simulink model "Miss_Sim_MatrixPilot"  (Simulink 7.0)
settings: Solver=ode1  SolverMode=SingleTasking  StartTime=0.0  StopTime=120  FixedStep=0.00025  MaxStep=0.01  MinStep=0.000001  RelTol=1e-12  AbsTol=1e-12
values from neighbouring files (symbols this model uses):
  alpha = [-180.     -90.        -5.         0.         5.        10.        15.        90.       180.       ]    [Miss_Data.m]
  Bref = 1.4    [Miss_Data.m]
  Clail = [ 0.         0.         0.         0.         0.         0.         0.         0.         0.       ]    [Miss_Data.m]
  Clp = [-0.5000    -0.5000    -0.496303  -0.494610  -0.492441  -0.492625  -0.522141  -0.5000    -0.5000   ]    [Miss_Data.m]
  Clr = [ 0.         0.         0.064175   0.123689   0.182593   0.241565   0.304725   0.         0.       ]    [Miss_Data.m]
  Clrud = [-0.000045  -0.000045  -0.000051  -0.000049  -0.000047  -0.000043  -0.000039  -0.000045  -0.000045 ]    [Miss_Data.m]
  Clv = [ 0.         0.        -0.098934  -0.137639  -0.176627  -0.217863  -0.281334   0.         0.       ]    [Miss_Data.m]
  Cmele = [-0.0180    -0.0180    -0.019125  -0.019236  -0.019052  -0.018576  -0.017796  -0.0180    -0.0180   ]    [Miss_Data.m]
  Cmq = [-12.3     -12.3      -12.288971 -12.358734 -12.331396 -12.223111 -12.072741 -12.3      -12.3      ]    [Miss_Data.m]
  Cmtot = [ 0.         2.         0.097340   0.036740  -0.047230  -0.137480  -0.110880  -2.         0.       ]    [Miss_Data.m]
  Cnail = [ 0.         0.         0.         0.         0.         0.         0.         0.         0.       ]    [Miss_Data.m]
  Cnp = [ 0.         0.         0.027830  -0.031473  -0.087981  -0.137950  -0.158851   0.         0.       ]    [Miss_Data.m]
  Cnr = [ 0.         0.        -0.041684  -0.040009  -0.043373  -0.056062  -0.120565   0.         0.       ]    [Miss_Data.m]
  Cnrud = [ 0.         0.         0.000628   0.000668   0.000698   0.000717   0.000725   0.         0.       ]    [Miss_Data.m]
  Cnv = [ 0.         0.         0.011072   0.000612  -0.009401  -0.018785  -0.019172   0.         0.       ]    [Miss_Data.m]
  Cref = 0.20    (= 0.2)    [Miss_Data.m]
  CROSS_TRACK = 1    [MatrixPilot_Parameters.m]
  CXq = [ 0.         0.        -0.507981  -0.147630   0.201483   0.570203   1.026474   0.         0.       ]    [Miss_Data.m]
  CXtot = [ 0.03       0.        -0.060470  -0.054540   0.003010   0.075240  -0.109550   0.         0.03     ]    [Miss_Data.m]
  CYp = [ 0.         0.        -0.217329  -0.145848  -0.074905  -0.009210   0.015572   0.         0.       ]    [Miss_Data.m]
  CYr = [ 0.         0.         0.049134   0.076782   0.103755   0.129584   0.152004   0.         0.       ]    [Miss_Data.m]
  CYrud = [-0.0016    -0.0016    -0.001484  -0.001575  -0.001641  -0.001681  -0.001693  -0.0016    -0.0016   ]    [Miss_Data.m]
  CYv = [ 0.         0.        -0.204296  -0.201289  -0.208918  -0.263073  -0.644029   0.         0.       ]    [Miss_Data.m]
  CZele = [-0.0067    -0.0067    -0.006924  -0.006962  -0.006897  -0.006734  -0.006498  -0.0067    -0.0067   ]    [Miss_Data.m]
  CZq = [ 0.         0.        -9.116849  -8.745556  -8.332987  -7.894125  -7.541102   0.         0.       ]    [Miss_Data.m]
  CZtot = [ 0.        10.         0.102580  -0.382550  -0.864940  -1.339340  -1.876430 -10.         0.       ]    [Miss_Data.m]
  DH = 10.    (= 10)    [MatrixPilot_Parameters.m]
  ele_damping = 0.7    [Miss_Data.m]
  ele_def_max = 30.    (= 30)    [Miss_Data.m]
  ele_frequency = 150.    (= 150)    [Miss_Data.m]
  ele_rate_limit = 285.    (= 285)    [Miss_Data.m]
  Ixx = 0.03004    [Miss_Data.m]
  Ixy = 0.    (= 0)    [Miss_Data.m]
  Ixz = 0.00137    [Miss_Data.m]
  Iyx = Ixy    (= 0)    [Miss_Data.m]
  Iyy = 0.01916    [Miss_Data.m]
  Iyz = 0.    (= 0)    [Miss_Data.m]
  Izx = Ixz    (= 0.00137)    [Miss_Data.m]
  Izy = Iyz    (= 0)    [Miss_Data.m]
  Izz = 0.04573    [Miss_Data.m]
  Mass = 0.950    (= 0.95)    [Miss_Data.m]
  rud_damping = 0.7    [Miss_Data.m]
  rud_def_max = 30.    (= 30)    [Miss_Data.m]
  rud_frequency = 150.    (= 150)    [Miss_Data.m]
  rud_rate_limit = 285.    (= 285)    [Miss_Data.m]
  SPEED_CONTROL = 1    [MatrixPilot_Parameters.m]
  Sref = 0.28    [Miss_Data.m]
  T_max = 1.    (= 1)    [MatrixPilot_Parameters.m]
  T_min = 0.35    [MatrixPilot_Parameters.m]
  Tdgps = 1.    (= 1)    [Miss_Data.m]
  theta_0 = -15.    (= -15)    [MatrixPilot_Parameters.m]
  theta_max = 15.    (= 15)    [MatrixPilot_Parameters.m]
  theta_min = -15.    (= -15)    [MatrixPilot_Parameters.m]
  Tmax = 10.    (= 10)    [Miss_Data.m]
  Vsp = 10.    (= 10)    [MatrixPilot_Parameters.m]
  WAYPOINT_RADIUS = 30.    (= 30)    [MatrixPilot_Parameters.m]
undefined symbols (not defined in the file or in its folder): F, MIL, Moderate
libraries: simulink x41, simulink_extras x26, dspstat3 x2, aerospace x1, aerolibanim x1, aerolibwind2 x1
(part 2 of 2)

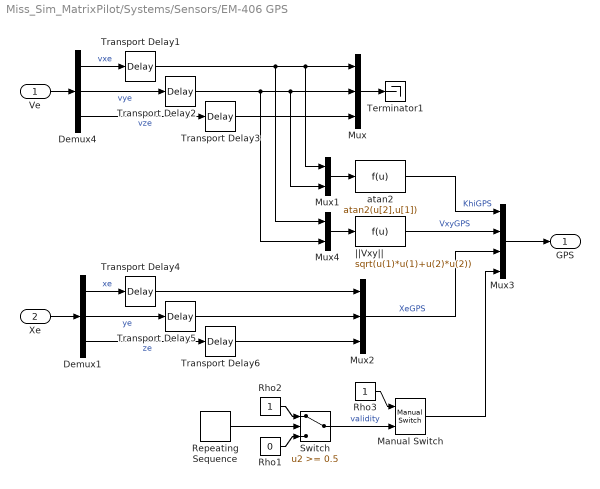
== system Miss_Sim_MatrixPilot/Systems/Sensors/EM-406 GPS ==
  Ve : Inport
  Xe : Inport  Port=2
  Demux1 : Demux  Outputs=3
  Demux4 : Demux  Outputs=3
  Manual Switch : simulink/Signal Routing/Manual Switch  SystemSampleTime=-1  sw=1  action=0  varsize=off
  Mux : Mux  Inputs=3
  Mux1 : Mux  Inputs=2
  Mux2 : Mux  Inputs=3
  Mux3 : Mux
  Mux4 : Mux  Inputs=2
  Repeating Sequence : simulink/Sources/Repeating Sequence  SystemSampleTime=-1  rep_seq_t="[0   120   120.001    140.  140.001  5000]"  rep_seq_y="[1    1       0           0        1          1]"
  Rho1 : Constant  Value=0
  Rho2 : Constant
  Rho3 : Constant
  Switch : Switch  Threshold=0.5  OutDataType=sfix(16)  OutScaling=2^0
  Terminator1 : Terminator
  Transport Delay1 : TransportDelay  DelayTime=Tdgps  InitialOutput=8.  BufferSize=4096
  Transport Delay{2..5} (4 alike) : TransportDelay  DelayTime=Tdgps  BufferSize=4096
  Transport Delay6 : TransportDelay  DelayTime=Tdgps  InitialOutput=-75  BufferSize=4096
  atan2 : Fcn  Expr=atan2(u[2],u[1])
  ||Vxy|| : Fcn  Expr=sqrt(u(1)*u(1)+u(2)*u(2))
  GPS : Outport
  wires:
  Transport Delay6/1 -> Mux2/3
  Transport Delay5/1 -> Mux2/2
  Transport Delay4/1 -> Mux2/1
  Transport Delay3/1 -> Mux/3
  Transport Delay2/1 -> Mux1/2, Mux/2, Mux4/2
  Transport Delay1/1 -> Mux1/1, Mux/1, Mux4/1
  Rho3/1 -> Manual Switch/1
  Manual Switch/1 -> Mux3/4
  Switch/1 -> Manual Switch/2  "validity"
  Repeating Sequence/1 -> Switch/2
  Rho2/1 -> Switch/1
  Rho1/1 -> Switch/3
  Mux3/1 -> GPS/1
  ||Vxy||/1 -> Mux3/2  "VxyGPS"
  Mux4/1 -> ||Vxy||/1
  Demux1/3 -> Transport Delay6/1  "ze"
  Xe/1 -> Demux1/1
  Mux2/1 -> Mux3/3  "XeGPS"
  Demux1/2 -> Transport Delay5/1  "ye"
  Demux1/1 -> Transport Delay4/1  "xe"
  Demux4/3 -> Transport Delay3/1  "vze"
  atan2/1 -> Mux3/1  "KhiGPS"
  Mux1/1 -> atan2/1
  Ve/1 -> Demux4/1
  Mux/1 -> Terminator1/1
  Demux4/2 -> Transport Delay2/1  "vye"
  Demux4/1 -> Transport Delay1/1  "vxe"

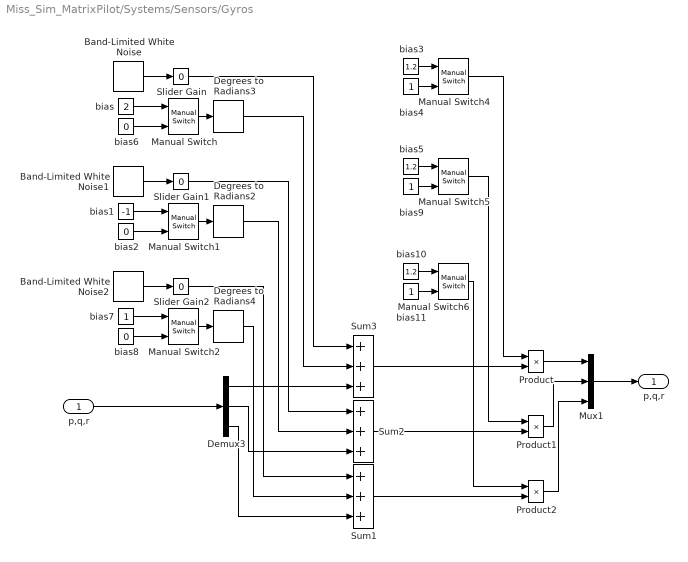
== system Miss_Sim_MatrixPilot/Systems/Sensors/Gyros ==
  p,q,r : Inport
  Band-Limited White Noise : simulink/Sources/Band-Limited White Noise  SystemSampleTime=-1  Cov=[0.000001]  Ts=0.01  seed=[23341]
  Band-Limited White Noise1 : simulink/Sources/Band-Limited White Noise  SystemSampleTime=-1  Cov=[0.000001]  Ts=0.01  seed=[23341]
  Band-Limited White Noise2 : simulink/Sources/Band-Limited White Noise  SystemSampleTime=-1  Cov=[0.000001]  Ts=0.01  seed=[23341]
  Degrees to Radians2 : simulink_extras/Transformations/Degrees to Radians  SystemSampleTime=-1
  Degrees to Radians3 : simulink_extras/Transformations/Degrees to Radians  SystemSampleTime=-1
  Degrees to Radians4 : simulink_extras/Transformations/Degrees to Radians  SystemSampleTime=-1
  Demux3 : Demux  Outputs=3
  Manual Switch{,1..2,4..6} (6 alike) : simulink/Signal Routing/Manual Switch  SystemSampleTime=-1  sw=0  action=0  varsize=off
  Mux1 : Mux  Inputs=3
  Product : Product  SaturateOnIntegerOverflow=on  RndMeth=Zero  InputSameDT=on
  Product1 : Product  SaturateOnIntegerOverflow=on  RndMeth=Zero  InputSameDT=on
  Product2 : Product  SaturateOnIntegerOverflow=on  RndMeth=Zero  InputSameDT=on
  Slider Gain : simulink/Math Operations/Slider Gain  SystemSampleTime=-1  low=0  gain=0  high=2
  Slider Gain1 : simulink/Math Operations/Slider Gain  SystemSampleTime=-1  low=0  gain=0  high=2
  Slider Gain2 : simulink/Math Operations/Slider Gain  SystemSampleTime=-1  low=0  gain=0  high=2
  Sum1 : Sum  Inputs=+++  SaturateOnIntegerOverflow=on  InputSameDT=on
  Sum2 : Sum  Inputs=+++  SaturateOnIntegerOverflow=on  InputSameDT=on
  Sum3 : Sum  Inputs=+++  SaturateOnIntegerOverflow=on  InputSameDT=on
  bias : Constant  Value=2  VectorParams1D=off
  bias1 : Constant  Value=-1  VectorParams1D=off
  bias10 : Constant  Value=1.2  VectorParams1D=off
  bias{4,7,9,11} (4 alike) : Constant  VectorParams1D=off
  bias2 : Constant  Value=0  VectorParams1D=off
  bias3 : Constant  Value=1.2  VectorParams1D=off
  bias5 : Constant  Value=1.2  VectorParams1D=off
  bias6 : Constant  Value=0  VectorParams1D=off
  bias8 : Constant  Value=0  VectorParams1D=off
  "p,q,r " : Outport
  wires:
  Mux1/1 -> "p,q,r "/1
  p,q,r/1 -> Demux3/1
  Band-Limited White Noise/1 -> Slider Gain/1
  Demux3/3 -> Sum1/3
  Demux3/2 -> Sum2/3
  Demux3/1 -> Sum3/3
  Band-Limited White Noise1/1 -> Slider Gain1/1
  Band-Limited White Noise2/1 -> Slider Gain2/1
  Slider Gain2/1 -> Sum1/1
  Slider Gain1/1 -> Sum2/1
  Slider Gain/1 -> Sum3/1
  Sum3/1 -> Product/2
  Product/1 -> Mux1/1
  Sum2/1 -> Product1/2
  Product1/1 -> Mux1/2
  Sum1/1 -> Product2/2
  Product2/1 -> Mux1/3
  Manual Switch4/1 -> Product/1
  Manual Switch6/1 -> Product2/1
  Manual Switch5/1 -> Product1/1
  Degrees to Radians3/1 -> Sum3/2
  Degrees to Radians2/1 -> Sum2/2
  Degrees to Radians4/1 -> Sum1/2
  Manual Switch/1 -> Degrees to Radians3/1
  bias/1 -> Manual Switch/1
  bias6/1 -> Manual Switch/2
  bias1/1 -> Manual Switch1/1
  bias2/1 -> Manual Switch1/2
  bias7/1 -> Manual Switch2/1
  bias8/1 -> Manual Switch2/2
  Manual Switch2/1 -> Degrees to Radians4/1
  Manual Switch1/1 -> Degrees to Radians2/1
  bias3/1 -> Manual Switch4/1
  bias4/1 -> Manual Switch4/2
  bias5/1 -> Manual Switch5/1
  bias9/1 -> Manual Switch5/2
  bias10/1 -> Manual Switch6/1
  bias11/1 -> Manual Switch6/2

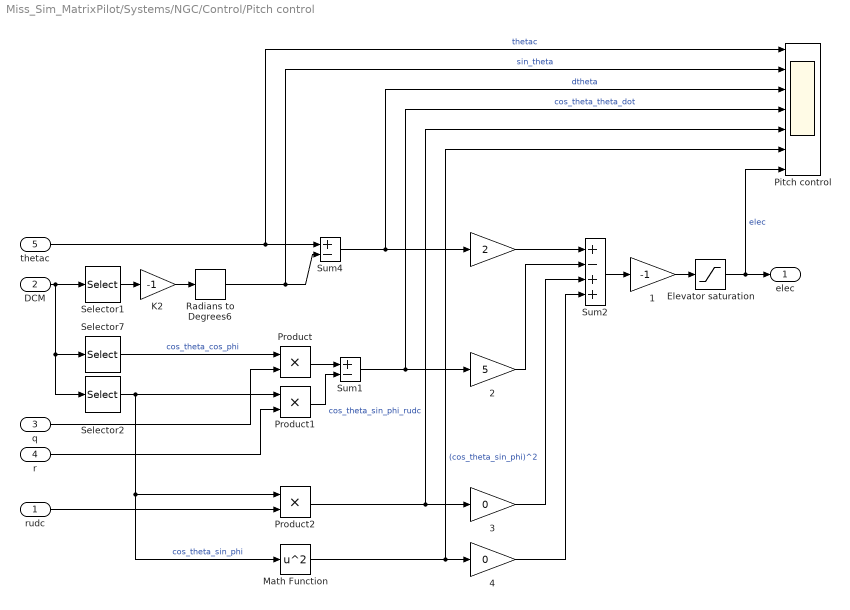
== system Miss_Sim_MatrixPilot/Systems/NGC/Control/Pitch control ==
  rudc : Inport
  DCM : Inport  Port=2
  q : Inport  Port=3
  r : Inport  Port=4
  thetac : Inport  Port=5
  " " : Gain  Gain=2  SaturateOnIntegerOverflow=on
  " 1" : Gain  Gain=-1  SaturateOnIntegerOverflow=on
  " 2" : Gain  Gain=5  SaturateOnIntegerOverflow=on
  " 3" : Gain  Gain=0  SaturateOnIntegerOverflow=on
  " 4" : Gain  Gain=0  SaturateOnIntegerOverflow=on
  Elevator saturation : Saturate  UpperLimit=ele_def_max  LowerLimit=-ele_def_max  OutDataType=sfix(16)  OutScaling=2^0
  K2 : Gain  Gain=-1  SaturateOnIntegerOverflow=on
  Math Function : Math  Operator=square  OutDataType=sfix(16)  OutScaling=2^0  SaturateOnIntegerOverflow=on
  Pitch control : Scope  NumInputPorts=7
      settings: TimeRange=20  YMin=0~-2~-3~-0.3~-1~-1~-5  YMax=5~5~5~0.6~1~1~3  SaveName=ScopeData13  MaxDataPoints=600000  Decimation=10  SampleInput=on
  Product : Product  OutDataType=sfix(16)  OutScaling=2^0  RndMeth=Zero
  Product1 : Product  OutDataType=sfix(16)  OutScaling=2^0  RndMeth=Zero
  Product2 : Product  OutDataType=sfix(16)  OutScaling=2^0  RndMeth=Zero
  Radians to Degrees6 : simulink_extras/Transformations/Radians to Degrees  SystemSampleTime=-1
  Selector1 : Selector  InputPortWidth=9  IndexOptions=Index vector (dialog)  Indices=7  OutputSizes=1
  Selector2 : Selector  InputPortWidth=9  IndexOptions=Index vector (dialog)  Indices=8  OutputSizes=1
  Selector7 : Selector  InputPortWidth=9  IndexOptions=Index vector (dialog)  Indices=9  OutputSizes=1
  Sum1 : Sum  Inputs=+-  SaturateOnIntegerOverflow=on  InputSameDT=on
  Sum2 : Sum  Inputs=+-++  SaturateOnIntegerOverflow=on  InputSameDT=on
  Sum4 : Sum  Inputs=+-  SaturateOnIntegerOverflow=on  InputSameDT=on
  elec : Outport
  wires:
  thetac/1 -> Sum4/1, Pitch control/1  "thetac"
  Sum4/1 -> Pitch control/3, " "/1  "dtheta"
  Sum2/1 -> " 1"/1
  Elevator saturation/1 -> elec/1, Pitch control/7  "elec"
  " 1"/1 -> Elevator saturation/1
  Selector1/1 -> K2/1
  K2/1 -> Radians to Degrees6/1
  Radians to Degrees6/1 -> Sum4/2, Pitch control/2  "sin_theta"
  q/1 -> Product/2
  Selector7/1 -> Product/1  "cos_theta_cos_phi"
  Selector2/1 -> Product1/1, Product2/1, Math Function/1  "cos_theta_sin_phi"
  r/1 -> Product1/2
  Product/1 -> Sum1/1
  Product1/1 -> Sum1/2
  Sum1/1 -> Pitch control/4, " 2"/1  "cos_theta_theta_dot"
  " 2"/1 -> Sum2/2
  rudc/1 -> Product2/2
  Product2/1 -> " 3"/1, Pitch control/5  "cos_theta_sin_phi_rudc"
  " 3"/1 -> Sum2/3
  Math Function/1 -> " 4"/1, Pitch control/6  "(cos_theta_sin_phi)^2"
  " 4"/1 -> Sum2/4
  DCM/1 -> Selector7/1, Selector2/1, Selector1/1
  " "/1 -> Sum2/1

== system Miss_Sim_MatrixPilot/Systems/NGC/Control/Yaw control ==
  note: bank angle response:
      | 29
      | 8
      | 7
      | 18
  yawc : Inport
  DCM : Inport  Port=2
  p : Inport  Port=3
  r : Inport  Port=4
  Bank control : Scope  NumInputPorts=5
      settings: TimeRange=15  YMin=-75~-40~-60~-40~-30  YMax=75~30~50~40~30  SaveName=ScopeData14  MaxDataPoints=600000  Decimation=10  SampleInput=on  SampleTime=0.025
  KDPHIP : Gain  Gain=29  SaturateOnIntegerOverflow=on
  KDPHIP1 : Gain  Gain=7  SaturateOnIntegerOverflow=on
  KDPHIP2 : Gain  Gain=50  SaturateOnIntegerOverflow=on
  KDPHIP3 : Gain  Gain=8  SaturateOnIntegerOverflow=on
  Radians to Degrees{1..3,6} (4 alike) : simulink_extras/Transformations/Radians to Degrees  SystemSampleTime=-1
  Rudder saturation : Saturate  UpperLimit=rud_def_max  LowerLimit=-rud_def_max  OutDataType=sfix(16)  OutScaling=2^0
  Selector : Selector  InputPortWidth=9  IndexOptions=Index vector (dialog)  Indices=8  OutputSizes=1
  Sum1 : Sum  Inputs=+---  SaturateOnIntegerOverflow=on  InputSameDT=on
  rudc : Outport
  wires:
  KDPHIP/1 -> Sum1/1
  Sum1/1 -> Rudder saturation/1
  p/1 -> KDPHIP1/1, Radians to Degrees2/1  "p"
  KDPHIP1/1 -> Sum1/3
  KDPHIP2/1 -> Sum1/4
  r/1 -> KDPHIP2/1, Radians to Degrees3/1  "r"
  KDPHIP3/1 -> Sum1/2
  DCM/1 -> Selector/1
  Radians to Degrees6/1 -> Bank control/1  "yawc (°)"
  Radians to Degrees1/1 -> Bank control/2  "phi (°)"
  Radians to Degrees2/1 -> Bank control/3  "p (°/s)"
  Radians to Degrees3/1 -> Bank control/4  "r (°/s)"
  yawc/1 -> KDPHIP/1, Radians to Degrees6/1  "yawc"
  Selector/1 -> KDPHIP3/1, Radians to Degrees1/1  "cos_theta_sin_phi"
  Rudder saturation/1 -> rudc/1, Bank control/5  "rudc (°)"

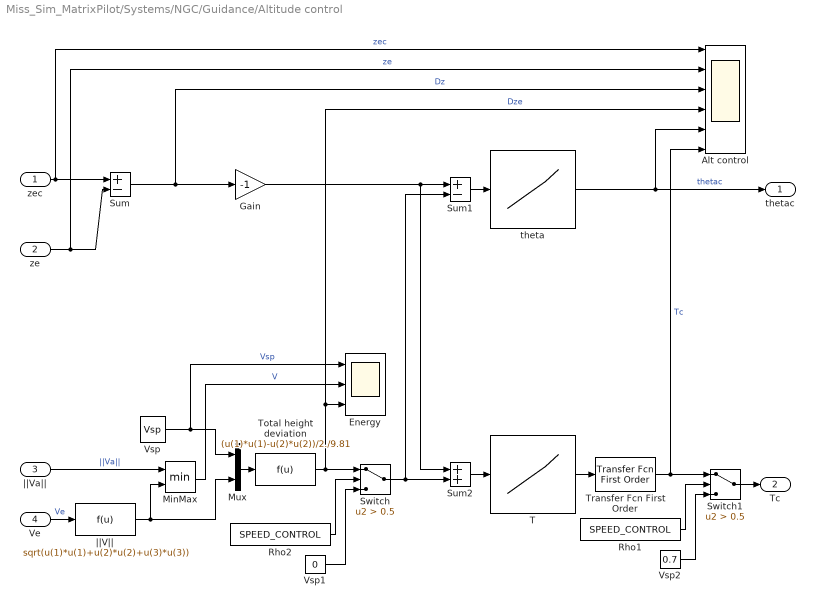
== system Miss_Sim_MatrixPilot/Systems/NGC/Guidance/Altitude control ==
  zec : Inport
  ze : Inport  Port=2
  ||Va|| : Inport  Port=3
  Ve : Inport  Port=4
  Alt control : Scope  NumInputPorts=6
      settings: TimeRange=40  YMin=-75~-79~2.25~-4.75~-2~0.435  YMax=-75~-77.25~4~-2.75~3.5~0.47  SaveName=ScopeData15  MaxDataPoints=600000  Decimation=10  SampleInput=on  SampleTime=0.025
  Energy : Scope  NumInputPorts=3
      settings: TimeRange=30  YMin=10.5~10.5~6.65  YMax=12.25~12.25~7.35  SaveName=ScopeData11  MaxDataPoints=600000  Decimation=10  SampleInput=on
  Gain : Gain  Gain=-1  ParameterDataType=sfix(16)  ParameterScaling=2^0  OutDataType=sfix(16)  OutScaling=2^0
  MinMax : MinMax  Inputs=2  OutDataType=sfix(16)  OutScaling=2^0
  Mux : Mux  Inputs=2
  Rho1 : Constant  Value=SPEED_CONTROL
  Rho2 : Constant  Value=SPEED_CONTROL
  Sum : Sum  Inputs=+-  SaturateOnIntegerOverflow=on  InputSameDT=on
  Sum1 : Sum  Inputs=+-  SaturateOnIntegerOverflow=on  InputSameDT=on
  Sum2 : Sum  SaturateOnIntegerOverflow=on  InputSameDT=on
  Switch : Switch  Criteria=u2 > Threshold  Threshold=0.5  OutDataType=sfix(16)  OutScaling=2^0
  Switch1 : Switch  Criteria=u2 > Threshold  Threshold=0.5  OutDataType=sfix(16)  OutScaling=2^0
  T : Lookup  InputValues="[-50  -DH  (-DH+0.001)  DH  50]"  Table="[0  0  T_min  T_max  T_max]"  SaturateOnIntegerOverflow=on
  Total height deviation : Fcn  Expr=(u(1)*u(1)-u(2)*u(2))/2./9.81
  Transfer Fcn First Order : simulink/Discrete/Transfer Fcn First Order  SystemSampleTime=-1  PoleZ=0.9375  ICPrevOutput=0.7  DoSatur=off
  Vsp : Constant  Value=Vsp
  Vsp1 : Constant  Value=0
  Vsp2 : Constant  Value=0.7
  theta : Lookup  InputValues="[-50  -DH  (-DH+0.001)  DH  50]"  Table="[theta_0  theta_0  theta_min  theta_max  theta_max]"  SaturateOnIntegerOverflow=on
  "||V|| " : Fcn  Expr=sqrt(u(1)*u(1)+u(2)*u(2)+u(3)*u(3))
  thetac : Outport
  Tc : Outport  Port=2
  wires:
  Ve/1 -> "||V|| "/1  "Ve"
  Vsp/1 -> Mux/1, Energy/1  "Vsp"
  MinMax/1 -> Energy/2  "V"
  Mux/1 -> Total height deviation/1
  Total height deviation/1 -> Switch/1, Alt control/4, Energy/3  "Dze"
  zec/1 -> Sum/1, Alt control/1  "zec"
  ze/1 -> Sum/2, Alt control/2  "ze"
  Sum/1 -> Alt control/3, Gain/1  "Dz"
  Sum2/1 -> T/1
  Sum1/1 -> theta/1
  T/1 -> Transfer Fcn First Order/1
  theta/1 -> thetac/1, Alt control/5  "thetac"
  Transfer Fcn First Order/1 -> Switch1/1, Alt control/6  "Tc"
  Gain/1 -> Sum1/1, Sum2/1
  Switch/1 -> Sum2/2, Sum1/2
  Rho2/1 -> Switch/2
  Vsp1/1 -> Switch/3
  ||Va||/1 -> MinMax/1  "||Va||"
  Switch1/1 -> Tc/1
  Vsp2/1 -> Switch1/3
  Rho1/1 -> Switch1/2
  "||V|| "/1 -> MinMax/2, Mux/2

== system Miss_Sim_MatrixPilot/Systems/NGC/Guidance/Heading control ==
  psic : Inport
  DCM : Inport  Port=2
  Embedded MATLAB Function : Stateflow chart  Description=toto
  Heading control : Scope  NumInputPorts=4
      settings: TimeRange=15  YMin=0~0~-50~-0.5  YMax=100~100~100~1  SaveName=ScopeData16  MaxDataPoints=600000  Decimation=10
  Mux : Mux  Inputs=2
  Radians to Degrees1 : simulink_extras/Transformations/Radians to Degrees  SystemSampleTime=-1
  Radians to Degrees6 : simulink_extras/Transformations/Radians to Degrees  SystemSampleTime=-1
  Selector : Selector  InputPortWidth=9  IndexOptions=Index vector (dialog)  Indices=4  OutputSizes=1
  Selector1 : Selector  InputPortWidth=9  IndexOptions=Index vector (dialog)  Indices=1  OutputSizes=1
  Sum1 : Sum  Inputs=+-  SaturateOnIntegerOverflow=on  InputSameDT=on
  Trigonometric Function : Trigonometry  Operator=cos
  Trigonometric Function1 : Trigonometry
  atans(y,x) : Fcn  Expr=atan2(u(2),u(1))
  yawc : Outport
  wires:
  Embedded MATLAB Function/1(yawc) -> yawc/1, Heading control/4  "yawc"
  psic/1 -> Trigonometric Function/1, Trigonometric Function1/1, Radians to Degrees1/1  "phic"
  Trigonometric Function/1 -> Embedded MATLAB Function/1(cos_psic)
  Trigonometric Function1/1 -> Embedded MATLAB Function/2(sin_psic)
  Selector1/1 -> Mux/1, Embedded MATLAB Function/3(cos_theta_cos_psi)
  Selector/1 -> Mux/2, Embedded MATLAB Function/4(cos_theta_sin_psi)
  Mux/1 -> atans(y,x)/1
  atans(y,x)/1 -> Radians to Degrees6/1
  Radians to Degrees6/1 -> Heading control/2, Sum1/2  "psi (°)"
  DCM/1 -> Selector/1, Selector1/1
  Radians to Degrees1/1 -> Heading control/1, Sum1/1  "phic (°)"
  Sum1/1 -> Heading control/3  "dpsi (°)"

== matlab function Systems/NGC/Guidance/Heading control/Embedded MATLAB Function ==
  data: yawc output inherited; cos_psic input inherited; sin_psic input inherited; cos_theta_cos_psi input inherited; cos_theta_sin_psi input inherited
%===============================================================================
function yawc = fcn(cos_psic, sin_psic, cos_theta_cos_psi, cos_theta_sin_psi)
%===============================================================================
% Navigation : computation of the steering command
%===============================================================================
dot_product   = cos_psic * cos_theta_cos_psi + sin_psic * cos_theta_sin_psi ;
cross_product = cos_theta_cos_psi * sin_psic - cos_theta_sin_psi * cos_psic ;

if dot_product < 0. 
   if cross_product > 0.
       yawc = 1. ;
   else
       yawc = -1 ;
   end
else
   yawc = cross_product ;
end

== matlab function Systems/NGC/Navigation/Embedded MATLAB Function ==
  data: debug output inherited; CROSS_TRACK input inherited; WAYPOINT_RADIUS input inherited; We input inherited; Vaxy input inherited; psic output inherited; zec output inherited; Xe input inherited
%===============================================================================
function [ debug, psic, zec ] = fcn( CROSS_TRACK, WAYPOINT_RADIUS, We, Vaxy, Xe )
%===============================================================================
% Navigation : computation of the commanded heading and altitude
%===============================================================================
% Waypoints
persistent WP_index
persistent WP_last_index
persistent Xe_init

if isempty( WP_index )
    WP_index = 1 ;
    WP_last_index = 0 ;
    Xe_init = [ Xe(1) Xe(2) Xe(3) ] ;
end

%WP.x = [ 50. 100. 150. 500.] ;
%WP.y = [  0.   0.   0.   0.] ;
%WP.y = [  0.  325.   0.  325.   0.  325. ] ;
%WP.x = [100.  100. 125.  125. 150.  150.] ;
WP.y = [107. -107. -107.  107. ] ;
WP.x = [ 45.   45.  -45.  -45. ] ;
%WP.y = [ 90.  -90.  -90.   90. ] ;
%WP.x = [ 100.   100.  -100.  -100. ] ;
%WP.y = [ 100.  -100.  -100.   100. ] ;
%WP.z = [-75.  -75. -75.  -75. -75. -75.] ;
WP.z = [-75.  -75.  -75.  -75. ] ;
%WP.z = [-75.  -75.  -125.  -125. ] ;
%WP.z = [-50.  -50.  -75.  -75. ] ;
WP.N = 4 ;

CTMARGIN = 32. ;

toPoint.x = WP.x(WP_index) ;
toPoint.y = WP.y(WP_index) ;
toPoint.z = WP.z(WP_index) ;

if WP_last_index == 0
    fromPoint.x = Xe_init(1) ;
    fromPoint.y = Xe_init(2) ;
    fromPoint.z = Xe_init(3) ;
else
    fromPoint.x = WP.x(WP_last_index) ;
    fromPoint.y = WP.y(WP_last_index) ;
    fromPoint.z = WP.z(WP_last_index) ;
end ;    

togoal.x = toPoint.x - Xe(1) ;
togoal.y = toPoint.y - Xe(2) ;

courseLeg.x = toPoint.x - fromPoint.x ;
courseLeg.y = toPoint.y - fromPoint.y ;

courseLeg.theta = 0. ;
courseLeg.theta = atan2( courseLeg.y, courseLeg.x ) ;

goal.costheta = cos( courseLeg.theta ) ;
goal.sintheta = sin( courseLeg.theta ) ;

tofinish_line = togoal.x * goal.costheta + togoal.y * goal.sintheta ;

% Cross track navigation
% ======================
if CROSS_TRACK == 1
    crosstrack = togoal.x * goal.sintheta - togoal.y * goal.costheta ;
    
    if abs(crosstrack) < CTMARGIN
        delta_khic = - crosstrack * 45. / CTMARGIN ;
    else
        delta_khic = - sign( crosstrack ) * 45. ;
    end ;
    
    if     delta_khic >  45.
        delta_khic =  45. ;
    elseif delta_khic < -45. 
        delta_khic = -45. ;
    end ;

    debug = crosstrack ;
 
    % Desired course over ground
    khic = pi()*delta_khic/180. + courseLeg.theta ;
    
% Standard navigation
% ===================
else
    % Desired course over ground
    khic = atan2( togoal.y, togoal.x ) ;

    debug = 0. ;
end;

% Desired heading
% ===============
% Account for the cross wind
% Compute the wind component that is perpendicular to the desired course
crossWind = We(1)*sin( khic ) - We(2)*cos( khic ) ;

if Vaxy > abs( crossWind )
   % the correction to the course is the arcsine of the ratio of cross 
   % wind to air speed
   psic = khic + asin( crossWind / Vaxy ) ;
else
   psic = khic ;
end;

% Altitude set point
% ==================
zec = toPoint.z ;

% Test finish line
% ================
if tofinish_line < WAYPOINT_RADIUS
    WP_last_index = WP_index ;
    
    if WP_index == WP.N WP_index = 1 ; 
    else WP_index = WP_index + 1 ;
    end ;
end ;
